simulink model "CompassCartBox"  (R2013b)
settings: Solver=ode3  SolverMode=SingleTasking  StartTime=0.0  StopTime=inf  RelTol=1e-3
PreLoadFcn:
  | TS = 0.1;
  | kp = 5; % motor proportional control constant
  | Kp_turn = 1;
  | MinSeg_Parameters
  | magXbias	= -27.850358;
  | magZbias	= -65.539659;
  | magXgain	= 0.013988;
  | magZgain	= 0.014555;
  | RSTime = [0.0 10.0 20.0 20.5 21.0 21.5 22.0 22.5 23.0 23.5 24.0 24.5 25.0 35.0 35.5 36.0 36.5 37.0 37.5 38.0 38.5 39.0 39.5 40.0 50.0 50.5 51.0 51.5 52.0 52.5 53.0 53.5 54.0 54.5 55.0 65.0 65.5 66.0 66.5 67.0 67.5 68.0 68.5 69.0 69.5 70.0 80.0];
  | RSHeading = [-2.9415926535897929e+00 -2.9415926535897929e+00 -2.9415926535897929e+00 -2.7845130209103033e+00 -2.6274333882308136e+00 -2.4703537555513240e+00 -2.3132741228718343e+00 -2.1561944901923447e+00 -1.9991148575128550e+00 -1.8420352248333653e+00 -1.6849555921538757e+00 -1.5278759594743860e+00 -1.3707963267948964e+00 -1.3707963267948964e+00 -1.2137166941154067e+00 -1.0566370614359171e+00 -8.9955742875642741e-01 -7.4247779607693776e-01 -5.8539816339744810e-01 -4.2831853071795845e-01 -2.7123889803846879e-01 -1.1415926535897913e-01 4.2920367320510522e-02 2.0000000000000018e-01 2.0000000000000018e-01 3.5707963267948983e-01 5.1415926535897949e-01 6.7123889803846915e-01 8.2831853071795880e-01 9.8539816339744846e-01 1.1424777960769381e+00 1.2995574287564278e+00 1.4566370614359174e+00 1.6137166941154071e+00 1.7707963267948967e+00 1.7707963267948967e+00 1.9278759594743864e+00 2.0849555921538760e+00 2.2420352248333657e+00 2.3991148575128554e+00 2.5561944901923450e+00 2.7132741228718347e+00 2.8703537555513243e+00 3.0274333882308140e+00 3.1845130209103036e+00 3.3415926535897933e+00 3.3415926535897933e+00];
undefined symbols (not defined in the file or in its folder): MinSegParam
libraries: MinSegLibrary_V2 x9, simulink x2, arduinolib x1
settings Model: SimulationMode=external  ExtModeTrigDuration=2  Creator=jmodiset  LastModifiedBy=mvernacc
settings OptimizationCC: OptimizeModelRefInitCode=on  LifeSpan=1
settings DebuggingCC: SolverPrmCheckMsg=none
settings HardwareCC: ProdBitPerInt=16  ProdBitPerPointer=8  ProdIntDivRoundTo=Zero  ProdEndianess=LittleEndian  ProdWordSize=8  ProdHWDeviceType=Atmel->AVR
settings RTWCC: SystemTargetFile=realtime.tlc  GenerateMakefile=off  TemplateMakefile=realtime.tmf  Description=Run on Target Hardware  RTWVerbose=off  ProcessScript=realtime_make_rtw_hook
settings STFCustomTargetCC: TargetLibSuffix=.a  GenerateSampleERTMain=on  ERTCustomFileBanners=on  SupportNonInlinedSFcns=off  SupportVariableSizeSignals=on  MATLABClassNameForMDSCustomization=Simulink.SoftwareTarget.ERTCustomization  GRTInterface=off  SystemTargetFile=realtime.tlc
settings ERTTargetCC: CodeReplacementLibrary=ANSI_C  GenerateSampleERTMain=on  ParMdlRefBuildCompliant=off  CompOptLevelCompliant=off  ConcurrentExecutionCompliant=off  CombineOutputUpdateFcns=off  ERTFirstTimeCompliant=off  SupportContinuousTime=on  SupportVariableSizeSignals=on  ModelStepFunctionPrototypeControlCompliant=off  CPPClassGenCompliant=off  ExtModeTransport=3  ExtModeMexFile=ext_serial_win32_comm  ExtModeMexArgs=0 1 9600  InlinedParameterPlacement=NonHierarchical  ERTSrcFileBannerTemplate=realtime_code_template.cgt  ERTHdrFileBannerTemplate=realtime_code_template.cgt  ERTDataSrcFileTemplate=realtime_code_template.cgt  ERTDataHdrFileTemplate=realtime_code_template.cgt  ERTCustomFileTemplate=realtime_file_process.tlc

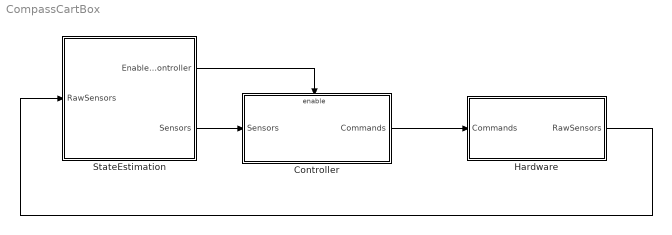
== system CompassCartBox ==
  Controller : Subsystem
  Hardware : Subsystem
  StateEstimation : Subsystem
  wires:
  Hardware/1(RawSensors) -> StateEstimation/1(RawSensors)
  StateEstimation/2(Sensors) -> Controller/1(Sensors)
  Controller/1(Commands) -> Hardware/1(Commands)
  StateEstimation/1(EnableController) -> Controller/Enable

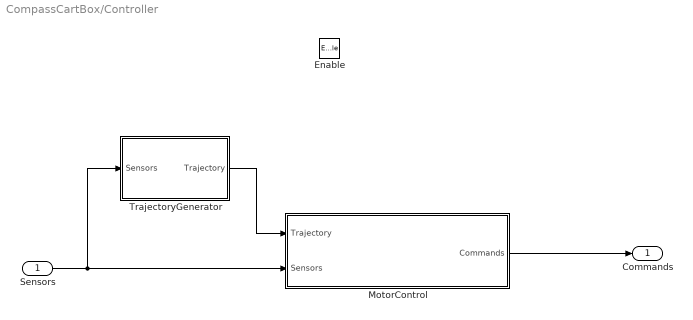
== system CompassCartBox/Controller ==
  Sensors : Inport
  Enable : EnablePort
  MotorControl : Subsystem
  TrajectoryGenerator : Subsystem
  Commands : Outport
  wires:
  Sensors/1 -> TrajectoryGenerator/1(Sensors), MotorControl/2(Sensors)
  TrajectoryGenerator/1(Trajectory) -> MotorControl/1(Trajectory)
  MotorControl/1(Commands) -> Commands/1

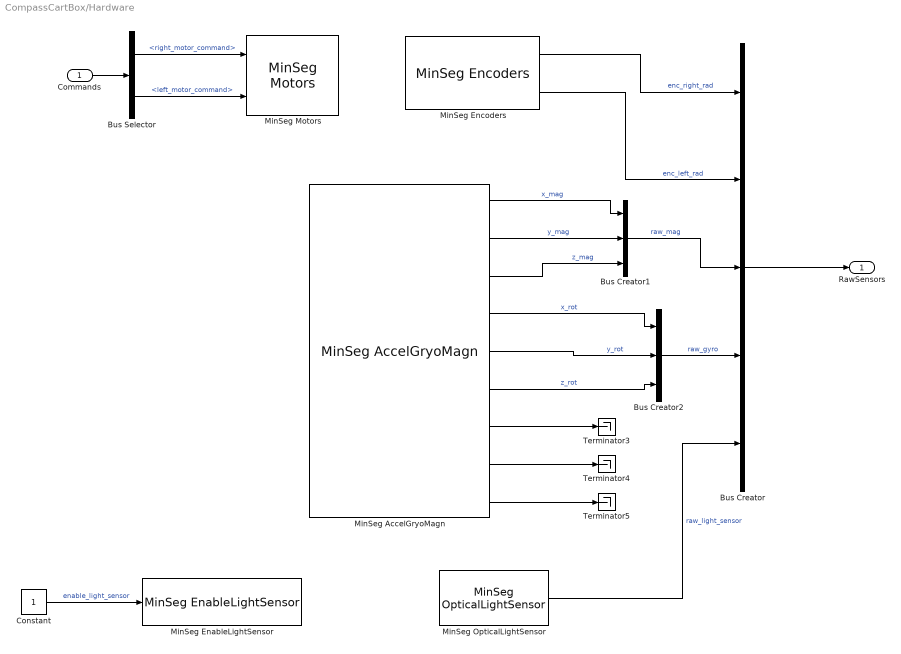
== system CompassCartBox/Hardware ==
  Commands : Inport
  Bus Creator : BusCreator  Inputs=5
  Bus Creator1 : BusCreator  Inputs=3
  Bus Creator2 : BusCreator  Inputs=3
  Bus Selector : BusSelector  OutputSignals=right_motor_command,left_motor_command
  Constant : Constant
  MinSeg AccelGryoMagn : MinSegLibrary_V2/MinSeg AccelGryoMagn  maskTS=TS
  MinSeg EnableLightSensor : MinSegLibrary_V2/MinSeg EnableLightSensor
  MinSeg Encoders : MinSegLibrary_V2/MinSeg Encoders  maskTS=TS
  MinSeg Motors : MinSegLibrary_V2/MinSeg Motors
  MinSeg OpticalLightSensor : MinSegLibrary_V2/MinSeg OpticalLightSensor  maskTS=TS
  Terminator3 : Terminator
  Terminator4 : Terminator
  Terminator5 : Terminator
  RawSensors : Outport
  wires:
  Commands/1 -> Bus Selector/1
  Bus Selector/1 -> MinSeg Motors/1  "<right_motor_command>"
  MinSeg Encoders/1 -> Bus Creator/1  "enc_right_rad"
  MinSeg Encoders/2 -> Bus Creator/2  "enc_left_rad"
  Bus Creator/1 -> RawSensors/1
  Bus Selector/2 -> MinSeg Motors/2  "<left_motor_command>"
  MinSeg AccelGryoMagn/4 -> Bus Creator2/1  "x_rot"
  MinSeg AccelGryoMagn/5 -> Bus Creator2/2  "y_rot"
  MinSeg AccelGryoMagn/6 -> Bus Creator2/3  "z_rot"
  MinSeg AccelGryoMagn/7 -> Terminator3/1
  MinSeg AccelGryoMagn/8 -> Terminator4/1
  MinSeg AccelGryoMagn/9 -> Terminator5/1
  MinSeg AccelGryoMagn/1 -> Bus Creator1/1  "x_mag"
  MinSeg AccelGryoMagn/2 -> Bus Creator1/2  "y_mag"
  MinSeg AccelGryoMagn/3 -> Bus Creator1/3  "z_mag"
  Bus Creator1/1 -> Bus Creator/3  "raw_mag"
  Bus Creator2/1 -> Bus Creator/4  "raw_gyro"
  MinSeg OpticalLightSensor/1 -> Bus Creator/5  "raw_light_sensor"
  Constant/1 -> MinSeg EnableLightSensor/1  "enable_light_sensor"

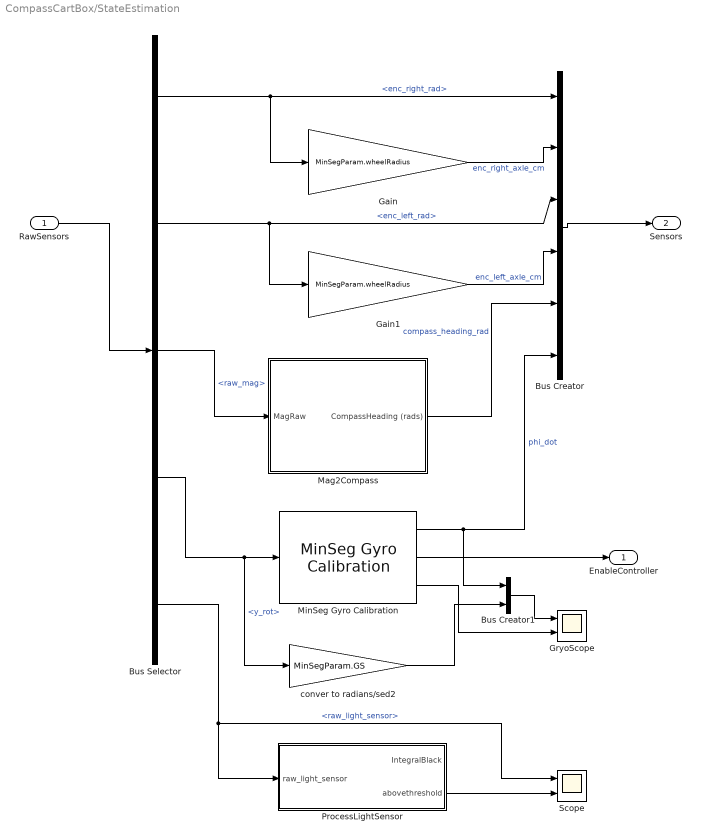
== system CompassCartBox/StateEstimation ==
  RawSensors : Inport
  Bus Creator : BusCreator  Inputs=6
  Bus Creator1 : BusCreator  Inputs=2
  Bus Selector : BusSelector  OutputSignals=enc_right_rad,enc_left_rad,raw_mag,raw_gyro.y_rot,raw_light_sensor
  Gain : Gain  Gain=MinSegParam.wheelRadius
  Gain1 : Gain  Gain=MinSegParam.wheelRadius
  GryoScope : Scope  NumInputPorts=2
      settings: YMin=-1.25~-0.00448989  YMax=2.75~-0.00448989  SaveName=GyroScopeData  MaxDataPoints=10000
  Mag2Compass : Subsystem
  MinSeg Gyro Calibration : MinSegLibrary_V2/MinSeg Gyro Calibration
  ProcessLightSensor : Subsystem
  Scope : Scope  NumInputPorts=2
      settings: YMin=250~0  YMax=650~1  SaveName=ScopeData2
  conver to radians/sed2 : Gain  Gain=MinSegParam.GS
  EnableController : Outport
  Sensors : Outport  Port=2
  wires:
  Bus Creator/1 -> Sensors/1
  Bus Selector/1 -> Gain/1, Bus Creator/1  "<enc_right_rad>"
  Bus Selector/2 -> Gain1/1, Bus Creator/3  "<enc_left_rad>"
  Gain/1 -> Bus Creator/2  "enc_right_axle_cm"
  RawSensors/1 -> Bus Selector/1
  Gain1/1 -> Bus Creator/4  "enc_left_axle_cm"
  Bus Selector/3 -> Mag2Compass/1(MagRaw)  "<raw_mag>"
  Mag2Compass/1(CompassHeading (rads)) -> Bus Creator/5  "compass_heading_rad"
  MinSeg Gyro Calibration/1 -> Bus Creator1/1, Bus Creator/6  "phi_dot"
  Bus Selector/4 -> conver to radians/sed2/1, MinSeg Gyro Calibration/1  "<y_rot>"
  MinSeg Gyro Calibration/2 -> EnableController/1
  Bus Selector/5 -> Scope/1, ProcessLightSensor/1(raw_light_sensor)  "<raw_light_sensor>"
  ProcessLightSensor/2(abovethreshold) -> Scope/2
  conver to radians/sed2/1 -> Bus Creator1/2
  Bus Creator1/1 -> GryoScope/1
  MinSeg Gyro Calibration/3 -> GryoScope/2

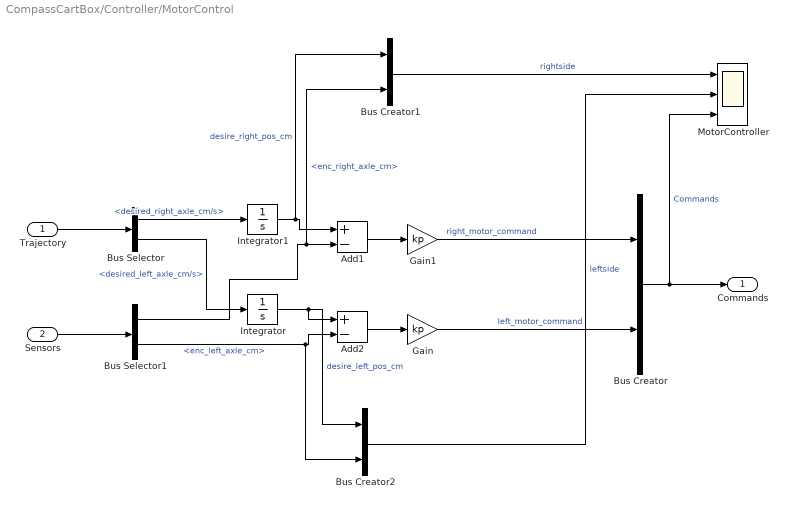
== system CompassCartBox/Controller/MotorControl ==
  Trajectory : Inport
  Sensors : Inport  Port=2
  Add1 : Sum  Inputs=+-
  Add2 : Sum  Inputs=+-
  Bus Creator : BusCreator  Inputs=2
  Bus Creator1 : BusCreator  Inputs=2
  Bus Creator2 : BusCreator  Inputs=2
  Bus Selector : BusSelector  OutputSignals=desired_right_axle_cm/s,desired_left_axle_cm/s
  Bus Selector1 : BusSelector  OutputSignals=enc_right_axle_cm,enc_left_axle_cm
  Gain : Gain  Gain=kp
  Gain1 : Gain  Gain=kp
  Integrator : Integrator
  Integrator1 : Integrator
  MotorController : Scope  NumInputPorts=3
      settings: TimeRange=10  YMin=-700~-700~0  YMax=800~800~650  SaveName=MCData
  Commands : Outport
  wires:
  Sensors/1 -> Bus Selector1/1
  Trajectory/1 -> Bus Selector/1
  Bus Creator/1 -> MotorController/3, Commands/1  "Commands"
  Gain/1 -> Bus Creator/2  "left_motor_command"
  Gain1/1 -> Bus Creator/1  "right_motor_command"
  Bus Selector/2 -> Integrator/1  "<desired_left_axle_cm/s>"
  Bus Selector/1 -> Integrator1/1  "<desired_right_axle_cm/s>"
  Bus Creator1/1 -> MotorController/1  "rightside"
  Bus Creator2/1 -> MotorController/2  "leftside"
  Bus Selector1/1 -> Bus Creator1/2, Add1/2  "<enc_right_axle_cm>"
  Bus Selector1/2 -> Bus Creator2/2, Add2/2  "<enc_left_axle_cm>"
  Integrator1/1 -> Bus Creator1/1, Add1/1  "desire_right_pos_cm"
  Integrator/1 -> Bus Creator2/1, Add2/1  "desire_left_pos_cm"
  Add1/1 -> Gain1/1
  Add2/1 -> Gain/1

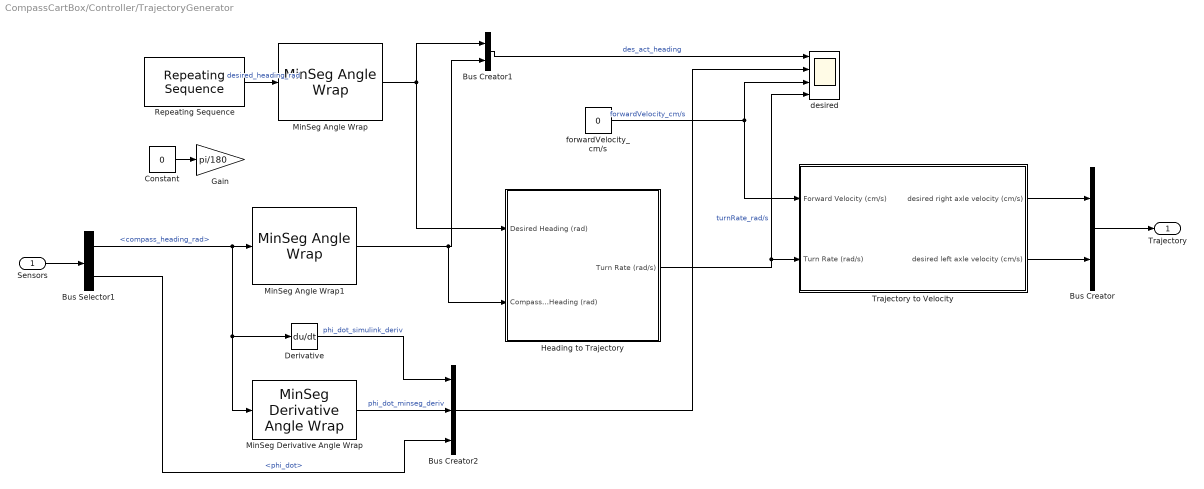
== system CompassCartBox/Controller/TrajectoryGenerator ==
  Sensors : Inport
  Bus Creator : BusCreator  Inputs=2
  Bus Creator1 : BusCreator  Inputs=2
  Bus Creator2 : BusCreator  Inputs=3
  Bus Selector1 : BusSelector  OutputSignals=compass_heading_rad,phi_dot
  Constant : Constant  Value=0
  Derivative : Derivative
  Gain : Gain  Gain=pi/180
  Heading to Trajectory : Subsystem
  MinSeg Angle Wrap : MinSegLibrary_V2/MinSeg Angle Wrap
  MinSeg Angle Wrap1 : MinSegLibrary_V2/MinSeg Angle Wrap
  MinSeg Derivative Angle Wrap : MinSegLibrary_V2/MinSeg Derivative Angle Wrap  daw_init_state=0  daw_ts=TS
  Repeating Sequence : simulink/Sources/Repeating Sequence  rep_seq_t=RSTime  rep_seq_y=RSHeading
  Trajectory to Velocity : Subsystem
  desired : Scope  NumInputPorts=4
      settings: TimeRange=10  YMin=-3.5~-1~-4.5~-5  YMax=3.5~1~2~5  SaveName=HeadingData
  forwardVelocity_cm/s : Constant  Value=0
  Trajectory : Outport
  wires:
  Heading to Trajectory/1(Turn Rate (rad/s)) -> desired/4, Trajectory to Velocity/2(Turn Rate (rad/s))  "turnRate_rad/s"
  Bus Creator/1 -> Trajectory/1
  forwardVelocity_cm/s/1 -> desired/3, Trajectory to Velocity/1(Forward Velocity (cm/s))  "forwardVelocity_cm/s"
  Trajectory to Velocity/1(desired right axle velocity (cm/s)) -> Bus Creator/1
  Trajectory to Velocity/2(desired left axle velocity (cm/s)) -> Bus Creator/2
  Sensors/1 -> Bus Selector1/1
  Bus Creator1/1 -> desired/1  "des_act_heading"
  Constant/1 -> Gain/1
  MinSeg Angle Wrap/1 -> Bus Creator1/1, Heading to Trajectory/1(Desired Heading (rad))
  MinSeg Angle Wrap1/1 -> Heading to Trajectory/2(Compass Heading (rad)), Bus Creator1/2
  Repeating Sequence/1 -> MinSeg Angle Wrap/1  "desired_heading_rad"
  Bus Selector1/1 -> MinSeg Angle Wrap1/1, Derivative/1, MinSeg Derivative Angle Wrap/1  "<compass_heading_rad>"
  Derivative/1 -> Bus Creator2/1  "phi_dot_simulink_deriv"
  MinSeg Derivative Angle Wrap/1 -> Bus Creator2/2  "phi_dot_minseg_deriv"
  Bus Selector1/2 -> Bus Creator2/3  "<phi_dot>"
  Bus Creator2/1 -> desired/2

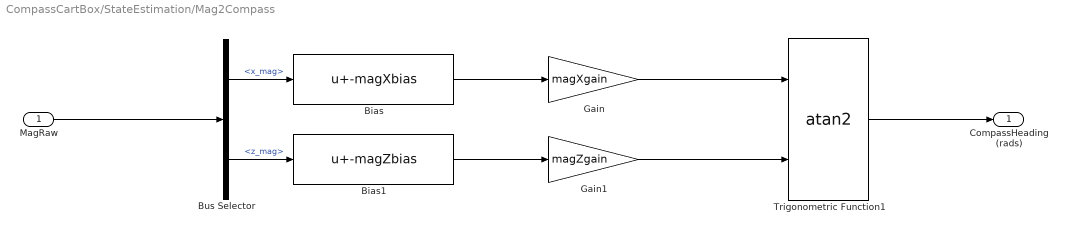
== system CompassCartBox/StateEstimation/Mag2Compass ==
  MagRaw : Inport
  Bias : Bias  Bias=-magXbias
  Bias1 : Bias  Bias=-magZbias
  Bus Selector : BusSelector  OutputSignals=x_mag,z_mag
  Gain : Gain  Gain=magXgain
  Gain1 : Gain  Gain=magZgain
  Trigonometric Function1 : Trigonometry  Operator=atan2
  CompassHeading (rads) : Outport
  wires:
  Bus Selector/2 -> Bias1/1  "<z_mag>"
  Bus Selector/1 -> Bias/1  "<x_mag>"
  Bias1/1 -> Gain1/1
  Bias/1 -> Gain/1
  Gain1/1 -> Trigonometric Function1/2
  Gain/1 -> Trigonometric Function1/1
  Trigonometric Function1/1 -> CompassHeading (rads)/1
  MagRaw/1 -> Bus Selector/1

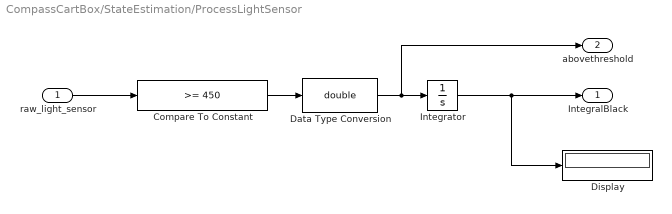
== system CompassCartBox/StateEstimation/ProcessLightSensor ==
  raw_light_sensor : Inport
  Compare To Constant : simulink/Logic and Bit Operations/Compare To Constant  relop=>=  const=450  OutDataTypeStr=uint8
  Data Type Conversion : DataTypeConversion  OutDataTypeStr=double
  Display : Display
  Integrator : Integrator
  IntegralBlack : Outport
  abovethreshold : Outport  Port=2
  wires:
  Integrator/1 -> IntegralBlack/1, Display/1
  raw_light_sensor/1 -> Compare To Constant/1
  Compare To Constant/1 -> Data Type Conversion/1
  Data Type Conversion/1 -> abovethreshold/1, Integrator/1

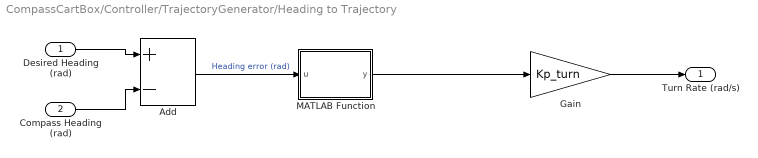
== system CompassCartBox/Controller/TrajectoryGenerator/Heading to Trajectory ==
  Desired Heading (rad) : Inport
  Compass Heading (rad) : Inport  Port=2
  Add : Sum  Inputs=+-
  Gain : Gain  Gain=Kp_turn
  MATLAB Function : MATLAB Function  TreatAsAtomicUnit=on
  Turn Rate (rad/s) : Outport
  wires:
  Desired Heading (rad)/1 -> Add/1
  Compass Heading (rad)/1 -> Add/2
  Add/1 -> MATLAB Function/1(u)  "Heading error (rad)"
  Gain/1 -> Turn Rate (rad/s)/1
  MATLAB Function/1(y) -> Gain/1

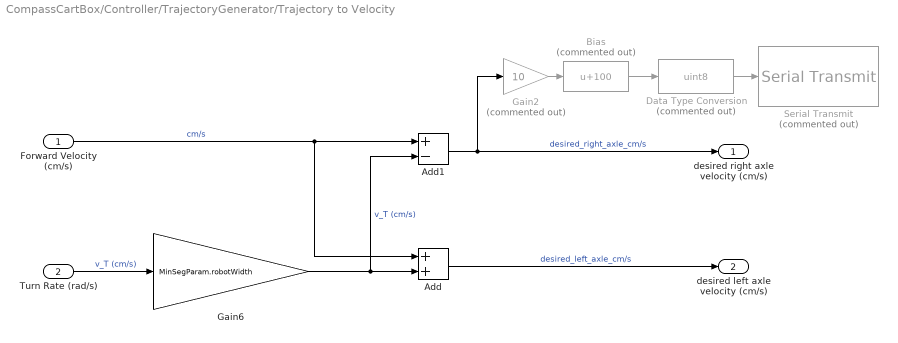
== system CompassCartBox/Controller/TrajectoryGenerator/Trajectory to Velocity ==
  Forward Velocity (cm/s) : Inport
  Turn Rate (rad/s) : Inport  Port=2
  Add : Sum
  Add1 : Sum  Inputs=+-
  Bias : Bias  Commented=on  Bias=100
  Data Type Conversion : DataTypeConversion  Commented=on  OutDataTypeStr=uint8
  Gain2 : Gain  Commented=on  Gain=10
  Gain6 : Gain  Gain=MinSegParam.robotWidth
  Serial Transmit : arduinolib/Serial Transmit  Commented=on  portNumber=0
  desired right axle velocity (cm/s) : Outport
  desired left axle velocity (cm/s) : Outport  Port=2
  wires:
  Forward Velocity (cm/s)/1 -> Add/1, Add1/1  "cm/s"
  Add/1 -> desired left axle velocity (cm/s)/1  "desired_left_axle_cm/s"
  Gain6/1 -> Add1/2, Add/2  "v_T (cm/s)"
  Turn Rate (rad/s)/1 -> Gain6/1  "v_T (cm/s)"
  Add1/1 -> Gain2/1, desired right axle velocity (cm/s)/1  "desired_right_axle_cm/s"
  Data Type Conversion/1 -> Serial Transmit/1
  Bias/1 -> Data Type Conversion/1
  Gain2/1 -> Bias/1

== matlab function CompassCartBox/Controller/TrajectoryGenerator/Heading to Trajectory/MATLAB Function ==
  data: u input; y output
function y = wrap_heading_error(u)
if u > pi
    y = u -2*pi;
elseif u <= -pi
    y = 2*pi + u;
else
    y = u;
end
end
